simulink model "carv_ident_simu"  (R2018a)
settings: Solver=VariableStepAuto  StartTime=0.0  StopTime=10.0  RelTol=1e-3
values from neighbouring files (symbols this model uses):
  Te = 1/800    (= 0.00125)    [RST_eleve.m]
settings Model: Creator=khennouh  LastModifiedBy=khennouh

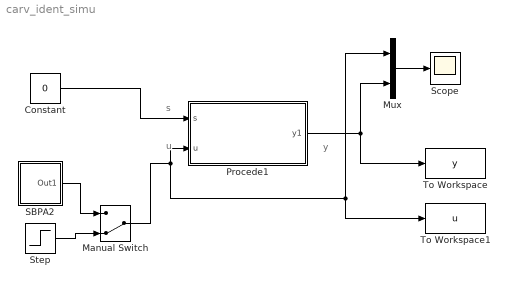
== system carv_ident_simu ==
  note: s
  note: u
  note: y
  Constant : Constant  Value=0
  Manual Switch : ManualSwitch  CurrentSetting=0
  Mux : Mux  Inputs=2
  Procede1 : Subsystem
      mask Display: disp('Procédé Simulé')
  SBPA2 : Subsystem  mask(Configuration d'une SBPA){A=5, Te=5, p=5, nr=5}
      mask prompts: A "Amplitude A"; Te "Sample Time Te=Ts"; p "Parameter p (frequency divisor)"; nr "Parameter nr (register length)"
      mask help:
      | A= amplitude du signal
      | p = diviseur de fréquence
      | nr = nbr de registres
      | Te = Sample Time (seconds)
      |
      | Pour plus de renseignements voir l'aide
      mask Help:
      | Cette SBPA est construite à l'aide de bloc discret en Z représentant des registres binaires.
      | L'aspect aléatoire des valeurs est obtenu par un modulo 2 entre certains bits de ce registre.
      mask Display: disp('SBPA')
  Scope : Scope
  Step : Step  Time=5  After=0  SampleTime=0
  To Workspace : ToWorkspace  VariableName=y  SampleTime=-1
  To Workspace1 : ToWorkspace  VariableName=u  SampleTime=-1
  wires:
  Mux/1 -> Scope/1
  Step/1 -> Manual Switch/2
  Procede1/1(y1) -> To Workspace/1, Mux/2
  SBPA2/1(Out1) -> Manual Switch/1
  Manual Switch/1 -> Mux/1, To Workspace1/1, Procede1/2(u)
  Constant/1 -> Procede1/1(s)

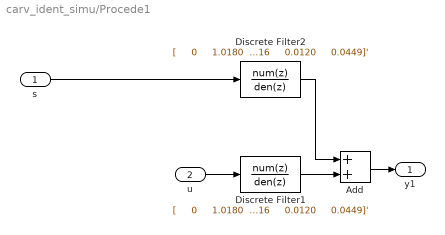
== system carv_ident_simu/Procede1 ==
  s : Inport
  u : Inport  Port=2
  Add : Sum
  Discrete Filter1 : DiscreteFilter  Numerator=|  Denominator=|  SampleTime=Te
      Numerator=|
      | [     0
      |     1.0180
      |    -2.1169
      |     0.6843
      |    -0.3008
      |     2.9943
      |    -3.0203
      |     0.8812
      |    -1.5539
      |     2.2356
      |    -0.7953
      |     0.6724
      |    -1.0735
      |     0.1364
      |     0.2454]'
      Denominator=|
      | [1.0000
      |    -1.7389
      |     1.0408
      |    -0.7931
      |     2.5618
      |    -2.8601
      |     1.7853
      |    -1.7239
      |     2.0897
      |    -1.2512
      |     1.0092
      |    -1.0000
      |     0.5016
      |     0.0120
      |     0.0449]'
  Discrete Filter2 : DiscreteFilter  Numerator=|  Denominator=|  SampleTime=Te
      Numerator=|
      | [     0
      |     1.0180
      |    -2.1169
      |     0.6843
      |    -0.3008
      |     2.9943
      |    -3.0203
      |     0.8812
      |    -1.5539
      |     2.2356
      |    -0.7953
      |     0.6724
      |    -1.0735
      |     0.1364
      |     0.2454]'
      Denominator=|
      | [1.0000
      |    -1.7389
      |     1.0408
      |    -0.7931
      |     2.5618
      |    -2.8601
      |     1.7853
      |    -1.7239
      |     2.0897
      |    -1.2512
      |     1.0092
      |    -1.0000
      |     0.5016
      |     0.0120
      |     0.0449]'
  y1 : Outport
  wires:
  s/1 -> Discrete Filter2/1
  u/1 -> Discrete Filter1/1
  Discrete Filter2/1 -> Add/1
  Discrete Filter1/1 -> Add/2
  Add/1 -> y1/1

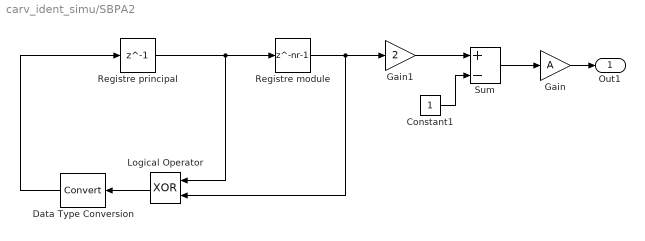
== system carv_ident_simu/SBPA2 ==
  Constant1 : Constant
  Data Type Conversion : DataTypeConversion  SampleTime=p*Te
  Gain : Gain  Gain=A  SaturateOnIntegerOverflow=on  OutDataTypeStr=Inherit: Same as input  ParamDataTypeStr=Inherit: Same as input
  Gain1 : Gain  Gain=2  SaturateOnIntegerOverflow=on  OutDataTypeStr=Inherit: Same as input  ParamDataTypeStr=Inherit: Same as input
  Logical Operator : Logic  Operator=XOR  AllPortsSameDT=off  OutDataTypeStr=boolean  SampleTime=p*Te
  Registre module : Delay  DelayLength=nr-1  InitialCondition=zeros(1,nr-1)  InputProcessing=Inherited  SampleTime=p*Te
  Registre principal : Delay  DelayLength=1  InitialCondition=1  InputProcessing=Inherited  SampleTime=p*Te
  Sum : Sum  Inputs=+-  SaturateOnIntegerOverflow=on  InputSameDT=on  OutDataTypeStr=Inherit: Same as first input
  Out1 : Outport
  wires:
  Registre module/1 -> Logical Operator/2, Gain1/1
  Registre principal/1 -> Registre module/1, Logical Operator/1
  Gain1/1 -> Sum/1
  Constant1/1 -> Sum/2
  Sum/1 -> Gain/1
  Gain/1 -> Out1/1
  Logical Operator/1 -> Data Type Conversion/1
  Data Type Conversion/1 -> Registre principal/1
